simulink model "EMPlanner_cs"  (R2020a)
settings: Solver=ode5  StartTime=0.0  StopTime=55  FixedStep=1/1000  RelTol=1e-3
PreLoadFcn:
  | mbxruntime.callbacks.PreLoadFcn(bdroot);
PostLoadFcn:
  | mbxruntime.callbacks.PostLoadFcn(bdroot);
InitFcn:
  | mbxruntime.callbacks.InitFcn(bdroot);
StartFcn:
  | mbxruntime.callbacks.StartFcn(bdroot);
StopFcn:
  | mbxruntime.callbacks.StopFcn(bdroot);
model workspace: external: MAT-File .\EMPlanner_cs_hws.mat (data not in the file)
values from neighbouring files (symbols this model uses):
  c_factor = 43.75    [emplanner_init.m]
  cf = -175016    [emplanner_init.m]
  control_predict_time = 0.01    [emplanner_init.m]
  cr = -130634    [emplanner_init.m]
  dp_col = 4    [emplanner_init.m]
  dp_row = 9    [emplanner_init.m]
  dp_sample_l = 1    [emplanner_init.m]
  dp_sample_s = 15    [emplanner_init.m]
  dp_w_obs = 1e8    (= 100000000)    [emplanner_init.m]
  dp_w_ref = 20    [emplanner_init.m]
  dp_w_smooth_dddl = 10000    [emplanner_init.m]
  dp_w_smooth_ddl = 2000    [emplanner_init.m]
  dp_w_smooth_dl = 300    [emplanner_init.m]
  KD_PID_distance = 0.0    (= 0)    [emplanner_init.m]
  KD_PID_speed = 0    [emplanner_init.m]
  KI_PID_distance = 0.0    (= 0)    [emplanner_init.m]
  KI_PID_speed = 0    [emplanner_init.m]
  KP_PID_distance = 0.5    [emplanner_init.m]
  KP_PID_speed = 1.8    [emplanner_init.m]
  la = 1.265    [emplanner_init.m]
  lb = 2.947-1.265    (= 1.682)    [emplanner_init.m]
  LQR_K1 = k(:,1)'    [emplanner_init.m]
  LQR_K2 = k(:,2)'    [emplanner_init.m]
  LQR_K3 = k(:,3)'    [emplanner_init.m]
  LQR_K4 = k(:,4)'    [emplanner_init.m]
  m = 2020    [emplanner_init.m]
  path_x = [7.7742 8.77358225507 9.77170536558 10.7685522493 11.7641171228 12.7583983581 13.7513958557 14.7431100776 15.7335416918 16.7226914411 17.7105600952 18.6971484329 ... (551 elements, 551x1)]    [test_path.mat]
  path_y = [-207.8202 -207.82020006 -207.820200616 -207.820202023 -207.82020429 -207.820207237 -207.820210603 -207.820214131 -207.82021762 -207.820220941 -207.820224011 -207.820226778 ... (551 elements, 551x1)]    [test_path.mat]
  qp_referenceline_w_length = 2    [emplanner_init.m]
  qp_referenceline_w_ref = 3    [emplanner_init.m]
  qp_referenceline_w_smooth = 1    [emplanner_init.m]
  qp_referenceline_x_lb = -0.2    [emplanner_init.m]
  qp_referenceline_x_ub = 0.2    [emplanner_init.m]
  qp_referenceline_y_lb = -0.2    [emplanner_init.m]
  qp_referenceline_y_ub = 0.2    [emplanner_init.m]
  rack_displacement = [-39.14 , -37.2 , -35.29 , -33.43 , -31.6 , -29.81 , -28.06 , -26.34 , -24.66 ,      -23.01 , -21.38 , -19.79 , -18.23 , -16.69 , -15.18 , -13.7 , -12.23 , -10.8 , -9.38 , -7.98 ,     -6.61 , -5.25 , -3.91 , -2.59 , -1.29 , 0 , 1.27 , 2.54 , 3.78 , 5.02 , 6.24 , 7.46 , 8.66 ,      9.86 , 11.05 , 12.24 , 13.41 , 14.59 , 15.76 , 16.92 , 18.09 , 19.25 , 20.42 , 21.59 , 22.76 ,      23.93 , 25.11 , 26 ...(+26 chars)    [emplanner_init.m]
  right_wheel_ground = [-70 ,-67.2 , -64.4 , -61.6 , -58.8 , -56 , -53.2 , -50.4 , -47.6 , -44.8 , -42 ,      -39.2 , -36.4 , -33.6 , -30.8 , -28 , -25.2 , -22.4 , -19.6 , -16.8 , -14 , -11.2 , -8.4 , -5.6 ,      -2.8 , 0 , 2.8 , 5.6 , 8.4 , 11.2 , 14 , 16.8 , 19.6 , 22.4 , 25.2 , 28 , 30.8 , 33.6 , 36.4 ,      39.2 , 42 , 44.8 , 47.6 , 50.4 , 53.2 , 56 , 58.8 , 61.6 , 64.4 , 67.2 , 70 ]    [emplanner_init.m]
  vx_break_point = zeros(1,5000)    [emplanner_init.m]
undefined symbols (not defined in the file or in its folder): aubr, DiscIntNeverNeededParam, tablebr, vubr, warningInitialVelocity, x0
libraries: simulink x19, PreScanSimulinkLibrary x12, simulink_extras x5, Solver_SF x1
(part 8 of 9)

== matlab function EMPlanner_cs/Audi_A8_Sedan_1/decision&planning module/EM Planner/MATLAB Function2 ==
  data: x_set_gcs input; match_point_index_set output; y_set_gcs input; path_x_set_gcs input; path_y_set_gcs input; path_heading_set_gcs input; path_kappa_set_gcs input; proj_point_x_set_gcs output; proj_point_y_set_gcs output; proj_point_heading_set_gcs output; proj_point_kappa_set_gcs output
function [match_point_index_set,proj_point_x_set_gcs,proj_point_y_set_gcs,proj_point_heading_set_gcs,...
    proj_point_kappa_set_gcs] = fcn(x_set_gcs,y_set_gcs,path_x_set_gcs,path_y_set_gcs,...
    path_heading_set_gcs,path_kappa_set_gcs)
% 该函数将批量计算点在给定路径下的匹配点编号和投影点信息   
% x_set_gcs,y_set_gcs 输入点信息集合
% path_x_set_gcs,path_y_set_gcs,path_heading_set_gcs,path_kappa_set_gcs 给定路径点信息集合
% match_point_index_set 匹配点编号集合
% proj_point_x_set_gcs,proj_point_y_set_gcs,proj_point_heading_set_gcs,proj_point_kappa_set_gcs 投影点信息集合

% 假设最多有181个点需要投影
n = 181;
% 对输出进行初始化
match_point_index_set = ones(n,1) *nan; 
proj_point_x_set_gcs = ones(n,1) *nan;  proj_point_y_set_gcs = ones(n,1) *nan;
proj_point_heading_set_gcs = ones(n,1) *nan;  proj_point_kappa_set_gcs = ones(n,1) *nan;

% 寻找匹配点时 需要利用上一个周期的结果 因此定义需要利用的静态变量
persistent is_first_run;
persistent pre_match_point_index_set;
persistent pre_path_x_set_gcs; persistent pre_path_y_set_gcs; % 通过上个周期匹配点位矢判断遍历方向
persistent pre_path_heading_set_gcs; persistent pre_path_kappa_set_gcs;
persistent pre_x_set_gcs; persistent pre_y_set_gcs; % 判断相邻帧检测的是否是同一个障碍物

if isempty(is_first_run)
    is_first_run = 0;
    % 首次运行 所有待求点都从给定路径路径第一个点开始找 往前遍历 且距离连续增长上限设为50
    for i = 1:length(x_set_gcs) % 存在的点都在前面 遍历到nan至后面的点都不存在
        if isnan(x_set_gcs(i))
            break;
        end
        start_find_index = 1; forward_stable_backward = 1; increase_count_limit = 50;
        % 计算匹配点编号
        match_point_index = CalMatchPointIndex(x_set_gcs(i),y_set_gcs(i),path_x_set_gcs,...
        path_y_set_gcs,path_heading_set_gcs,path_kappa_set_gcs,start_find_index,...
        increase_count_limit, forward_stable_backward);
        % 计算投影点信息
        [proj_point_x_gcs,proj_point_y_gcs,proj_point_heading_gcs,proj_point_kappa_gcs] = ...
        CalProjPointInfo(x_set_gcs(i),y_set_gcs(i),path_x_set_gcs,path_y_set_gcs,path_heading_set_gcs,...
        path_kappa_set_gcs,match_point_index);
        % 将每个点求解信息添加到集合
        match_point_index_set(i) = match_point_index;
        proj_point_x_set_gcs(i) = proj_point_x_gcs; proj_point_y_set_gcs(i) = proj_point_y_gcs;
        proj_point_heading_set_gcs(i) = proj_point_heading_gcs; 
        proj_point_kappa_set_gcs(i) = proj_point_kappa_gcs;
    end
    % 保存该周期信息 以便下周期使用
    pre_match_point_index_set = match_point_index_set;
    pre_path_x_set_gcs = path_x_set_gcs; pre_path_y_set_gcs = path_y_set_gcs;
    pre_path_heading_set_gcs = path_heading_set_gcs; pre_path_kappa_set_gcs = path_kappa_set_gcs;
    pre_x_set_gcs = x_set_gcs; pre_y_set_gcs = y_set_gcs;
else
    % 需要使用上周期信息
    for i = 1:length(x_set_gcs)
        if isnan(x_set_gcs(i))
            break;
        end
        % 检测相邻帧是否是同一物体求解
        dis = sqrt((x_set_gcs(i)-pre_x_set_gcs(i))^2 + (y_set_gcs(i)-pre_y_set_gcs(i))^2);
        if dis > 10  % 相邻帧(相隔0.1s)同一物体距离不可能这么大
            % 说明相邻帧不是同一物体 上周期该物体已经消失在车辆的检测范围内
            % 把上周期该物体匹配点编号信息清空
            pre_match_point_index_set(i) = nan;
        end
        if isnan(pre_match_point_index_set(i))
            % 说明该物体是第一次寻找匹配点 从头开始寻找 且往前遍历
            start_find_index = 1; forward_stable_backward = 1; increase_count_limit = 50;
        else
            % 说明该物体上周期已经寻找过匹配点  判断开始寻找编号 和遍历方向
            start_find_index = pre_match_point_index_set(i); increase_count_limit = 5;
            % 提取上周期匹配点信息
            pre_match_point_x = pre_path_x_set_gcs(pre_match_point_index_set(i));
            pre_match_point_y = pre_path_y_set_gcs(pre_match_point_index_set(i));
            pre_match_point_heading = pre_path_heading_set_gcs(pre_match_point_index_set(i));
            % 通过该物体上周期匹配点位置到本周期位置向量和上周期匹配点切向量的点乘来判断遍历方向
            vector_preMatch_current = [x_set_gcs(i),y_set_gcs(i)] - [pre_match_point_x, pre_match_point_y];
            vector_tor_preMatch = [cos(pre_match_point_heading), sin(pre_match_point_heading)];
            forward_stable_backward = dot(vector_preMatch_current, vector_tor_preMatch);
        end
        % 计算匹配点编号
        match_point_index = CalMatchPointIndex(x_set_gcs(i),y_set_gcs(i),path_x_set_gcs,...
        path_y_set_gcs,path_heading_set_gcs,path_kappa_set_gcs,start_find_index,...
        increase_count_limit, forward_stable_backward);
        % 计算投影点信息
        [proj_point_x_gcs,proj_point_y_gcs,proj_point_heading_gcs,proj_point_kappa_gcs] = ...
        CalProjPointInfo(x_set_gcs(i),y_set_gcs(i),path_x_set_gcs,path_y_set_gcs,path_heading_set_gcs,...
        path_kappa_set_gcs,match_point_index);
        % 将每个点求解信息添加到集合
        match_point_index_set(i) = match_point_index;
        proj_point_x_set_gcs(i) = proj_point_x_gcs; proj_point_y_set_gcs(i) = proj_point_y_gcs;
        proj_point_heading_set_gcs(i) = proj_point_heading_gcs; 
        proj_point_kappa_set_gcs(i) = proj_point_kappa_gcs;
    end
    % 保存该周期信息 以便下周期使用
    pre_match_point_index_set = match_point_index_set;
    pre_path_x_set_gcs = path_x_set_gcs; pre_path_y_set_gcs = path_y_set_gcs;
    pre_path_heading_set_gcs = path_heading_set_gcs; pre_path_kappa_set_gcs = path_kappa_set_gcs;
    pre_x_set_gcs = x_set_gcs; pre_y_set_gcs = y_set_gcs;
end
end

== matlab function EMPlanner_cs/Audi_A8_Sedan_1/decision&planning module/EM Planner/Cartesian2Frenet/MATLAB Function4 ==
  data: ax_set input; s_dot2_set output; ay_set input; proj_heading_set input; proj_kappa_set input; l_set input; s_dot_set input; dl_set input; l_dot2_set output; ddl_set output
function [s_dot2_set,l_dot2_set,ddl_set] = fcn(ax_set,ay_set,proj_heading_set,proj_kappa_set,l_set,s_dot_set,dl_set)
%由于不知道有多少个点需要做坐标转换，设一个最大值做缓冲
n = 128;
% 输出初始化
s_dot2_set = ones(n,1)*nan;
l_dot2_set = ones(n,1)*nan;
ddl_set = ones(n,1)*nan;

for i = 1:length(l_set)
    if isnan(l_set(i))
       break;
    end
    a_h = [ax_set(i);ay_set(i)];
    n_r = [-sin(proj_heading_set(i));cos(proj_heading_set(i))];
    t_r = [cos(proj_heading_set(i));sin(proj_heading_set(i))];
    %近似认为dkr/ds 为0 简化计算
    l_dot2_set(i) = a_h'*n_r - proj_kappa_set(i) * (1 - proj_kappa_set(i) * l_set(i)) * s_dot_set(i)^2;
    s_dot2_set(i) = (1/(1 - proj_kappa_set(i) * l_set(i)))* (a_h' * t_r + 2 * proj_kappa_set(i) * dl_set(i) * s_dot_set(i)^2);
    % 要考虑加速度为0的情况
    if (s_dot2_set(i) < 1e-6)
        ddl_set(i) = 0;
    else
        ddl_set(i) = (l_dot2_set(i) - dl_set(i)*s_dot2_set(i))/(s_dot_set(i)^2);
    end
end

== matlab function EMPlanner_cs/Audi_A8_Sedan_1/decision&planning module/EM Planner/increase DP path nodes1 ==
  data: plan_start_point_s_fcs input; dp_path_s_final_set_fcs output; plan_start_point_l_fcs input; plan_start_point_dl_fcs input; plan_start_point_ddl_fcs input; dp_path_s_init_set_fcs input; dp_path_l_init_set_fcs input; dp_path_l_final_set_fcs output; dp_path_dl_final_set_fcs output; dp_path_ddl_final_set_fcs output
function [dp_path_s_final_set_fcs,dp_path_l_final_set_fcs,dp_path_dl_final_set_fcs,dp_path_ddl_final_set_fcs] = ...
    fcn(plan_start_point_s_fcs,plan_start_point_l_fcs,plan_start_point_dl_fcs,plan_start_point_ddl_fcs,dp_path_s_init_set_fcs,dp_path_l_init_set_fcs)
% 原有的动态规划的路径点太少  该函数用来增密路径点
% 输入:plan_start_point_info_fcs 规划起点信息 dp_path_info_init_set_fcs 动态规划初始点集合信息
% 输出:dp_path_info_final_set_fcs 动态规划最终点集合信息
% 原有的动态规划的路径点太少  该函数用来增密原有的动态规划得到的初始路径点
% 通过原有的规划点进行增密
% 假设增密之后横向每隔一米踩一个点
ds = 1;
% 原来路径为 规划起点-> 动态规划点1 -> 动态规划点2 -> 动态规划点3 -> 动态规划点4 -> 动态规划点5
% 增密后路径为 规划起点->(新增点->新增点->新增点)->动态规划点1->(新增点->新增点->新增点)->动态规划点2->...
% 如 规划起点-> 动态规划点1 为一个五次多项式  通过ds取多项式多个点 即为新增的点

% 假设增密之后最多200个点
n = 200;
% 输出初始化
dp_path_s_final_set_fcs = ones(n,1)*nan;dp_path_l_final_set_fcs = ones(n,1)*nan;
dp_path_dl_final_set_fcs = ones(n,1)*nan; dp_path_ddl_final_set_fcs = ones(n,1)*nan;

% 第一个五次多项式的起点为规划起点
start_s = plan_start_point_s_fcs; start_l = plan_start_point_l_fcs; 
start_dl = plan_start_point_dl_fcs; start_ddl = plan_start_point_ddl_fcs;

s_cur = []; l_cur = []; dl_cur = []; ddl_cur = []; %开辟动态数组存储所有采样点

for i = 1:length(dp_path_s_init_set_fcs)
    if isnan(dp_path_s_init_set_fcs(i))
        break;   %点不存在 退出
    end
    s_temp = []; l_temp = []; dl_temp = []; ddl_temp = []; %开辟临时动态数组存储当前循环采样点
    % 对规划起点-> 动态规划点1 -> 动态规划点2 -> 动态规划点3 -> 动态规划点4 -> 动态规划点5->...进行采样
    for j = 1:10000  % 取个较大的循环 下面通过条件break退出循环就
        s_node = start_s + ds * (j-1);   %增密后各个采样点s坐标  l,dl,ddl需要通过五次多项式计算
        if s_node < dp_path_s_init_set_fcs(i)
            s_temp = [s_temp, s_node]; % 将满足条件的增密点添加进数组
        else
            break;
        end
    end
    % % 求出五次多项式终点的边界条件
    end_s = dp_path_s_init_set_fcs(i); end_l = dp_path_l_init_set_fcs(i); end_dl = 0; end_ddl = 0;
    [a0,a1,a2,a3,a4,a5] = CalQuinticCoeffient(start_s,start_l,start_dl,start_ddl,end_s,end_l,end_dl,end_ddl);
    % 通过五次多项式求出每个采样点的l,dl,ddl
    for k = 1:length(s_temp)
        l_node = a0 + a1 * s_temp(k) + a2 * s_temp(k)^2+ a3 * s_temp(k)^3 + a4 * s_temp(k)^4 + a5 * s_temp(k)^5;
        l_temp = [l_temp,l_node];
        dl_node = a1 + 2 * a2 * s_temp(k) + 3 * a3 * s_temp(k)^2 + 4 * a4 * s_temp(k)^3 + 5 * a5 * s_temp(k)^4;
        dl_temp = [dl_temp,dl_node];
        ddl_node = 2 * a2 + 6 * a3 * s_temp(k) + 12 * a4 * s_temp(k)^2 + 20 * a5 * s_temp(k)^3;
        ddl_temp = [ddl_temp, ddl_node];
    end 
    % 将当前循环记录的采样点信息记录到总的动态数组里
    s_cur = [s_cur, s_temp]; l_cur = [l_cur, l_temp]; dl_cur = [dl_cur, dl_temp]; ddl_cur = [ddl_cur, ddl_temp];           
     % end的值赋值给start 做下一步循环
    start_s = end_s;start_l = end_l;start_dl = end_dl;start_ddl = end_ddl;
end

for i = 1:length(s_cur)
    % 防止增密之后点的个数超过最大容量
    if i > n
        break;
    end
    % 保证s坐标严格单调上升
    dp_path_s_final_set_fcs(i) = plan_start_point_s_fcs + ds * (i - 1);
%     dp_path_s_final_set_fcs(i) = s_cur(i);
    dp_path_l_final_set_fcs(i) = l_cur(i);
    dp_path_dl_final_set_fcs(i) = dl_cur(i);
    dp_path_ddl_final_set_fcs(i) = ddl_cur(i);
end
end

== matlab function EMPlanner_cs/Audi_A8_Sedan_1/decision&planning module/EM Planner/obs/MATLAB Function3 ==
  data: x_set_gcs input; match_point_index_set output; y_set_gcs input; path_x_set_gcs input; path_y_set_gcs input; path_heading_set_gcs input; path_kappa_set_gcs input; proj_point_x_set_gcs output; proj_point_y_set_gcs output; proj_point_heading_set_gcs output; proj_point_kappa_set_gcs output
function [match_point_index_set,proj_point_x_set_gcs,proj_point_y_set_gcs,proj_point_heading_set_gcs,...
    proj_point_kappa_set_gcs] = fcn(x_set_gcs,y_set_gcs,path_x_set_gcs,path_y_set_gcs,...
    path_heading_set_gcs,path_kappa_set_gcs)
% 该函数将批量计算点在给定路径下的匹配点编号和投影点信息   
% x_set_gcs,y_set_gcs 输入点信息集合
% path_x_set_gcs,path_y_set_gcs,path_heading_set_gcs,path_kappa_set_gcs 给定路径点信息集合
% match_point_index_set 匹配点编号集合
% proj_point_x_set_gcs,proj_point_y_set_gcs,proj_point_heading_set_gcs,proj_point_kappa_set_gcs 投影点信息集合

% 假设最多有181个点需要投影
n = 181;
% 对输出进行初始化
match_point_index_set = ones(n,1) *nan; 
proj_point_x_set_gcs = ones(n,1) *nan;  proj_point_y_set_gcs = ones(n,1) *nan;
proj_point_heading_set_gcs = ones(n,1) *nan;  proj_point_kappa_set_gcs = ones(n,1) *nan;

% 寻找匹配点时 需要利用上一个周期的结果 因此定义需要利用的静态变量
persistent is_first_run;
persistent pre_match_point_index_set;
persistent pre_path_x_set_gcs; persistent pre_path_y_set_gcs; % 通过上个周期匹配点位矢判断遍历方向
persistent pre_path_heading_set_gcs; persistent pre_path_kappa_set_gcs;
persistent pre_x_set_gcs; persistent pre_y_set_gcs; % 判断相邻帧检测的是否是同一个障碍物

if isempty(is_first_run)
    is_first_run = 0;
    % 首次运行 所有待求点都从给定路径路径第一个点开始找 往前遍历 且距离连续增长上限设为50
    for i = 1:length(x_set_gcs) % 存在的点都在前面 遍历到nan至后面的点都不存在
        if isnan(x_set_gcs(i))
            break;
        end
        start_find_index = 1; forward_stable_backward = 1; increase_count_limit = 50;
        % 计算匹配点编号
        match_point_index = CalMatchPointIndex(x_set_gcs(i),y_set_gcs(i),path_x_set_gcs,...
        path_y_set_gcs,path_heading_set_gcs,path_kappa_set_gcs,start_find_index,...
        increase_count_limit, forward_stable_backward);
        % 计算投影点信息
        [proj_point_x_gcs,proj_point_y_gcs,proj_point_heading_gcs,proj_point_kappa_gcs] = ...
        CalProjPointInfo(x_set_gcs(i),y_set_gcs(i),path_x_set_gcs,path_y_set_gcs,path_heading_set_gcs,...
        path_kappa_set_gcs,match_point_index);
        % 将每个点求解信息添加到集合
        match_point_index_set(i) = match_point_index;
        proj_point_x_set_gcs(i) = proj_point_x_gcs; proj_point_y_set_gcs(i) = proj_point_y_gcs;
        proj_point_heading_set_gcs(i) = proj_point_heading_gcs; 
        proj_point_kappa_set_gcs(i) = proj_point_kappa_gcs;
    end
    % 保存该周期信息 以便下周期使用
    pre_match_point_index_set = match_point_index_set;
    pre_path_x_set_gcs = path_x_set_gcs; pre_path_y_set_gcs = path_y_set_gcs;
    pre_path_heading_set_gcs = path_heading_set_gcs; pre_path_kappa_set_gcs = path_kappa_set_gcs;
    pre_x_set_gcs = x_set_gcs; pre_y_set_gcs = y_set_gcs;
else
    % 需要使用上周期信息
    for i = 1:length(x_set_gcs)
        if isnan(x_set_gcs(i))
            break;
        end
        % 检测相邻帧是否是同一物体求解
        dis = sqrt((x_set_gcs(i)-pre_x_set_gcs(i))^2 + (y_set_gcs(i)-pre_y_set_gcs(i))^2);
        if dis > 10  % 相邻帧(相隔0.1s)同一物体距离不可能这么大
            % 说明相邻帧不是同一物体 上周期该物体已经消失在车辆的检测范围内
            % 把上周期该物体匹配点编号信息清空
            pre_match_point_index_set(i) = nan;
        end
        if isnan(pre_match_point_index_set(i))
            % 说明该物体是第一次寻找匹配点 从头开始寻找 且往前遍历
            start_find_index = 1; forward_stable_backward = 1; increase_count_limit = 50;
        else
            % 说明该物体上周期已经寻找过匹配点  判断开始寻找编号 和遍历方向
            start_find_index = pre_match_point_index_set(i); increase_count_limit = 5;
            % 提取上周期匹配点信息
            pre_match_point_x = pre_path_x_set_gcs(pre_match_point_index_set(i));
            pre_match_point_y = pre_path_y_set_gcs(pre_match_point_index_set(i));
            pre_match_point_heading = pre_path_heading_set_gcs(pre_match_point_index_set(i));
            % 通过该物体上周期匹配点位置到本周期位置向量和上周期匹配点切向量的点乘来判断遍历方向
            vector_preMatch_current = [x_set_gcs(i),y_set_gcs(i)] - [pre_match_point_x, pre_match_point_y];
            vector_tor_preMatch = [cos(pre_match_point_heading), sin(pre_match_point_heading)];
            forward_stable_backward = dot(vector_preMatch_current, vector_tor_preMatch);
        end
        % 计算匹配点编号
        match_point_index = CalMatchPointIndex(x_set_gcs(i),y_set_gcs(i),path_x_set_gcs,...
        path_y_set_gcs,path_heading_set_gcs,path_kappa_set_gcs,start_find_index,...
        increase_count_limit, forward_stable_backward);
        % 计算投影点信息
        [proj_point_x_gcs,proj_point_y_gcs,proj_point_heading_gcs,proj_point_kappa_gcs] = ...
        CalProjPointInfo(x_set_gcs(i),y_set_gcs(i),path_x_set_gcs,path_y_set_gcs,path_heading_set_gcs,...
        path_kappa_set_gcs,match_point_index);
        % 将每个点求解信息添加到集合
        match_point_index_set(i) = match_point_index;
        proj_point_x_set_gcs(i) = proj_point_x_gcs; proj_point_y_set_gcs(i) = proj_point_y_gcs;
        proj_point_heading_set_gcs(i) = proj_point_heading_gcs; 
        proj_point_kappa_set_gcs(i) = proj_point_kappa_gcs;
    end
    % 保存该周期信息 以便下周期使用
    pre_match_point_index_set = match_point_index_set;
    pre_path_x_set_gcs = path_x_set_gcs; pre_path_y_set_gcs = path_y_set_gcs;
    pre_path_heading_set_gcs = path_heading_set_gcs; pre_path_kappa_set_gcs = path_kappa_set_gcs;
    pre_x_set_gcs = x_set_gcs; pre_y_set_gcs = y_set_gcs;
end
end

== matlab function EMPlanner_cs/Audi_A8_Sedan_1/decision&planning module/EM Planner/obs/Cartesian2Frenet1/MATLAB Function ==
  data: x_set_gcs input; s_set_fcs output; y_set_gcs input; path_x_set_gcs input; path_y_set_gcs input; path_heading_set_gcs input; match_point_index_set input; proj_point_x_set_gcs input; proj_point_y_set_gcs input; proj_point_heading_set_gcs input; l_set_fcs output; matchPoint_index_s_set_fcs input
function [s_set_fcs,l_set_fcs] = fun(x_set_gcs,y_set_gcs,path_x_set_gcs,path_y_set_gcs,path_heading_set_gcs,match_point_index_set,...
    proj_point_x_set_gcs,proj_point_y_set_gcs,proj_point_heading_set_gcs,matchPoint_index_s_set_fcs)
% 将函数批量将给定点的(x,y)转化成(s,l)
% 假设最多有181个点需要转换坐标
n = 181;
% 输出初始化
s_set_fcs = ones(n,1)*nan; l_set_fcs = ones(n,1)*nan;
for i = 1:length(x_set_gcs)
    if isnan(x_set_gcs(i))
        break;
    end
    s_set_fcs(i) = CalSFromOriginPoint(matchPoint_index_s_set_fcs,path_x_set_gcs,path_y_set_gcs,path_heading_set_gcs,...
                                proj_point_x_set_gcs(i),proj_point_y_set_gcs(i),match_point_index_set(i));
    vector_rh = [x_set_gcs(i),y_set_gcs(i)];
    vector_rp = [proj_point_x_set_gcs(i),proj_point_y_set_gcs(i)];
    vector_np = [-sin(proj_point_heading_set_gcs(i)),cos(proj_point_heading_set_gcs(i))];
    l_set_fcs(i) = dot(vector_rh-vector_rp, vector_np);
end
end

== matlab function EMPlanner_cs/Audi_A8_Sedan_1/decision&planning module/referenceline provider/solve heading and kappa求解给定path的heading角和曲率 ==
  data: path_x_set_gcs output; path_y_set_gcs output; path_heading_set_gcs output; path_x_set_gcs input; path_y_set_gcs input; path_kappa_set_gcs output
function [path_x_set_gcs,path_y_set_gcs,path_heading_set_gcs,path_kappa_set_gcs] = fcn(path_x_set_gcs,path_y_set_gcs)
%该函数将计算全局路径的切线方向与x轴的夹角和曲率
%输入：path_x_set_gcs,path_y_set_gcs 给定路径坐标 都是列向量
%输出：path_heading_gcs path_kappa_gcs 给定路径的heading和曲率
%输出初始化
if isrow(path_x_set_gcs)
    path_x_set_gcs = path_x_set_gcs';   % 保证为列向量
    path_y_set_gcs = path_y_set_gcs';
end
[path_heading_set_gcs,path_kappa_set_gcs] = CalHeadingAndKappa(path_x_set_gcs,path_y_set_gcs);
end

== matlab function EMPlanner_cs/Audi_A8_Sedan_1/decision&planning module/referenceline provider/MATLAB Function6 ==
  data: x_set_gcs input; match_point_index_set output; y_set_gcs input; path_x_set_gcs input; path_y_set_gcs input; path_heading_set_gcs input; path_kappa_set_gcs input; proj_point_x_set_gcs output; proj_point_y_set_gcs output; proj_point_heading_set_gcs output; proj_point_kappa_set_gcs output
function [match_point_index_set,proj_point_x_set_gcs,proj_point_y_set_gcs,proj_point_heading_set_gcs,...
    proj_point_kappa_set_gcs] = fcn(x_set_gcs,y_set_gcs,path_x_set_gcs,path_y_set_gcs,...
    path_heading_set_gcs,path_kappa_set_gcs)
% 该函数将批量计算点在给定路径下的匹配点编号和投影点信息   
% x_set_gcs,y_set_gcs 输入点信息集合
% path_x_set_gcs,path_y_set_gcs,path_heading_set_gcs,path_kappa_set_gcs 给定路径点信息集合
% match_point_index_set 匹配点编号集合
% proj_point_x_set_gcs,proj_point_y_set_gcs,proj_point_heading_set_gcs,proj_point_kappa_set_gcs 投影点信息集合

% 假设最多有181个点需要投影
n = 181;
% 对输出进行初始化
match_point_index_set = ones(n,1) *nan; 
proj_point_x_set_gcs = ones(n,1) *nan;  proj_point_y_set_gcs = ones(n,1) *nan;
proj_point_heading_set_gcs = ones(n,1) *nan;  proj_point_kappa_set_gcs = ones(n,1) *nan;

% 寻找匹配点时 需要利用上一个周期的结果 因此定义需要利用的静态变量
persistent is_first_run;
persistent pre_match_point_index_set;
persistent pre_path_x_set_gcs; persistent pre_path_y_set_gcs; % 通过上个周期匹配点位矢判断遍历方向
persistent pre_path_heading_set_gcs; persistent pre_path_kappa_set_gcs;
persistent pre_x_set_gcs; persistent pre_y_set_gcs; % 判断相邻帧检测的是否是同一个障碍物

if isempty(is_first_run)
    is_first_run = 0;
    % 首次运行 所有待求点都从给定路径路径第一个点开始找 往前遍历 且距离连续增长上限设为50
    for i = 1:length(x_set_gcs) % 存在的点都在前面 遍历到nan至后面的点都不存在
        if isnan(x_set_gcs(i))
            break;
        end
        start_find_index = 1; forward_stable_backward = 1; increase_count_limit = 50;
        % 计算匹配点编号
        match_point_index = CalMatchPointIndex(x_set_gcs(i),y_set_gcs(i),path_x_set_gcs,...
        path_y_set_gcs,path_heading_set_gcs,path_kappa_set_gcs,start_find_index,...
        increase_count_limit, forward_stable_backward);
        % 计算投影点信息
        [proj_point_x_gcs,proj_point_y_gcs,proj_point_heading_gcs,proj_point_kappa_gcs] = ...
        CalProjPointInfo(x_set_gcs(i),y_set_gcs(i),path_x_set_gcs,path_y_set_gcs,path_heading_set_gcs,...
        path_kappa_set_gcs,match_point_index);
        % 将每个点求解信息添加到集合
        match_point_index_set(i) = match_point_index;
        proj_point_x_set_gcs(i) = proj_point_x_gcs; proj_point_y_set_gcs(i) = proj_point_y_gcs;
        proj_point_heading_set_gcs(i) = proj_point_heading_gcs; 
        proj_point_kappa_set_gcs(i) = proj_point_kappa_gcs;
    end
    % 保存该周期信息 以便下周期使用
    pre_match_point_index_set = match_point_index_set;
    pre_path_x_set_gcs = path_x_set_gcs; pre_path_y_set_gcs = path_y_set_gcs;
    pre_path_heading_set_gcs = path_heading_set_gcs; pre_path_kappa_set_gcs = path_kappa_set_gcs;
    pre_x_set_gcs = x_set_gcs; pre_y_set_gcs = y_set_gcs;
else
    % 需要使用上周期信息
    for i = 1:length(x_set_gcs)
        if isnan(x_set_gcs(i))
            break;
        end
        % 检测相邻帧是否是同一物体求解
        dis = sqrt((x_set_gcs(i)-pre_x_set_gcs(i))^2 + (y_set_gcs(i)-pre_y_set_gcs(i))^2);
        if dis > 10  % 相邻帧(相隔0.1s)同一物体距离不可能这么大
            % 说明相邻帧不是同一物体 上周期该物体已经消失在车辆的检测范围内
            % 把上周期该物体匹配点编号信息清空
            pre_match_point_index_set(i) = nan;
        end
        if isnan(pre_match_point_index_set(i))
            % 说明该物体是第一次寻找匹配点 从头开始寻找 且往前遍历
            start_find_index = 1; forward_stable_backward = 1; increase_count_limit = 50;
        else
            % 说明该物体上周期已经寻找过匹配点  判断开始寻找编号 和遍历方向
            start_find_index = pre_match_point_index_set(i); increase_count_limit = 5;
            % 提取上周期匹配点信息
            pre_match_point_x = pre_path_x_set_gcs(pre_match_point_index_set(i));
            pre_match_point_y = pre_path_y_set_gcs(pre_match_point_index_set(i));
            pre_match_point_heading = pre_path_heading_set_gcs(pre_match_point_index_set(i));
            % 通过该物体上周期匹配点位置到本周期位置向量和上周期匹配点切向量的点乘来判断遍历方向
            vector_preMatch_current = [x_set_gcs(i),y_set_gcs(i)] - [pre_match_point_x, pre_match_point_y];
            vector_tor_preMatch = [cos(pre_match_point_heading), sin(pre_match_point_heading)];
            forward_stable_backward = dot(vector_preMatch_current, vector_tor_preMatch);
        end
        % 计算匹配点编号
        match_point_index = CalMatchPointIndex(x_set_gcs(i),y_set_gcs(i),path_x_set_gcs,...
        path_y_set_gcs,path_heading_set_gcs,path_kappa_set_gcs,start_find_index,...
        increase_count_limit, forward_stable_backward);
        % 计算投影点信息
        [proj_point_x_gcs,proj_point_y_gcs,proj_point_heading_gcs,proj_point_kappa_gcs] = ...
        CalProjPointInfo(x_set_gcs(i),y_set_gcs(i),path_x_set_gcs,path_y_set_gcs,path_heading_set_gcs,...
        path_kappa_set_gcs,match_point_index);
        % 将每个点求解信息添加到集合
        match_point_index_set(i) = match_point_index;
        proj_point_x_set_gcs(i) = proj_point_x_gcs; proj_point_y_set_gcs(i) = proj_point_y_gcs;
        proj_point_heading_set_gcs(i) = proj_point_heading_gcs; 
        proj_point_kappa_set_gcs(i) = proj_point_kappa_gcs;
    end
    % 保存该周期信息 以便下周期使用
    pre_match_point_index_set = match_point_index_set;
    pre_path_x_set_gcs = path_x_set_gcs; pre_path_y_set_gcs = path_y_set_gcs;
    pre_path_heading_set_gcs = path_heading_set_gcs; pre_path_kappa_set_gcs = path_kappa_set_gcs;
    pre_x_set_gcs = x_set_gcs; pre_y_set_gcs = y_set_gcs;
end
end

== matlab function EMPlanner_cs/Audi_A8_Sedan_1/decision&planning module/EM Planner/Cartesian2Frenet/MATLAB Function1 ==
  data: l_set_fcs input; sdot_set_fcs output; vx_set_gcs input; vy_set_gcs input; proj_point_heading_set_gcs input; proj_point_kappa_set_gcs input; ldot_set_fcs output; dl_set_fcs output
function [sdot_set_fcs, ldot_set_fcs, dl_set_fcs] = fun(l_set_fcs,vx_set_gcs,vy_set_gcs,proj_point_heading_set_gcs,proj_point_kappa_set_gcs)
% 该函数批量转化坐标得到    sdot_set_fcs, ldot_set_fcs, dl_set_fcs
% 假设最多有181个点需要转换坐标
n = 181;
% 输出初始化
sdot_set_fcs = ones(n,1)*nan; ldot_set_fcs = ones(n,1)*nan; dl_set_fcs = ones(n,1)*nan;

for i = 1:length(vx_set_gcs)
    if isnan(vx_set_gcs(i))
        break;
    end
    vector_vh = [vx_set_gcs(i),vy_set_gcs(i)];
    vector_tp = [cos(proj_point_heading_set_gcs(i)),sin(proj_point_heading_set_gcs(i))];
    vector_np = [-sin(proj_point_heading_set_gcs(i)),cos(proj_point_heading_set_gcs(i))];
    sdot_set_fcs(i) = (dot(vector_vh,vector_tp)) / (1-proj_point_kappa_set_gcs(i)*l_set_fcs(i));
    ldot_set_fcs(i) = dot(vector_vh,vector_np);
    if abs(sdot_set_fcs(i)) < 1e-6
        dl_set_fcs(i) = 0;
    else
        dl_set_fcs(i) = ldot_set_fcs(i) / sdot_set_fcs(i);
    end
end
end

== matlab function EMPlanner_cs/Audi_A8_Sedan_1/decision&planning module/EM Planner/Cartesian2Frenet/MATLAB Function2 ==
  data: ax_set_gcs input; sdotdot_set_fcs output; ay_set_gcs input; proj_point_heading_set_gcs input; proj_point_kappa_set_gcs input; l_set_fcs input; sdot_set_fcs input; dl_set_fcs input; ldotdot_set_fcs output; ddl_set_fcs output
function [sdotdot_set_fcs, ldotdot_set_fcs, ddl_set_fcs] = fun(ax_set_gcs,ay_set_gcs,proj_point_heading_set_gcs,proj_point_kappa_set_gcs,...
    l_set_fcs, sdot_set_fcs,dl_set_fcs)
% 该函数批量转化坐标得到    sdotdot_set_fcs, ldotdot_set_fcs, ddl_set_fcs
% 假设最多有181个点需要转换坐标
n = 181;
% 输出初始化
sdotdot_set_fcs = ones(n,1)*nan; ldotdot_set_fcs = ones(n,1)*nan; ddl_set_fcs = ones(n,1)*nan;

for i = 1:length(ax_set_gcs)
    if isnan(ax_set_gcs(i))
        break;
    end
    vector_ah = [ax_set_gcs(i),ay_set_gcs(i)];
    vector_tp = [cos(proj_point_heading_set_gcs(i)),sin(proj_point_heading_set_gcs(i))];
    vector_np = [-sin(proj_point_heading_set_gcs(i)),cos(proj_point_heading_set_gcs(i))];
    sdotdot_set_fcs(i) = (dot(vector_ah,vector_tp) + 2*proj_point_kappa_set_gcs(i)*dl_set_fcs(i)*sdot_set_fcs(i)^2) / (1-proj_point_kappa_set_gcs(i)*l_set_fcs(i));
    ldotdot_set_fcs(i) = dot(vector_ah,vector_np) - proj_point_kappa_set_gcs(i) * (1-proj_point_kappa_set_gcs(i)*l_set_fcs(i)) * sdot_set_fcs(i)^2;
    if abs(sdotdot_set_fcs(i)) < 1e-6
        ddl_set_fcs(i) = 0;
    else
        ddl_set_fcs(i) = (ldotdot_set_fcs(i) - dl_set_fcs(i) * sdotdot_set_fcs(i)) / sdot_set_fcs(i)^2;
    end
end
end

== matlab function EMPlanner_cs/Audi_A8_Sedan_1/decision&planning module/EM Planner/obs/obs filter ==
  data: host_x_gcs input; obs_x_set_final_gcs output; host_y_gcs input; host_heading_gcs input; obs_x_set_gcs input; obs_y_set_gcs input; obs_velocity_set_gcs input; obs_velocity_heading_set_gcs input; obs_y_set_final_gcs output; obs_velocity_set_final_gcs output; obs_velocity_heading_set_final_gcs output
function [obs_x_set_final_gcs,obs_y_set_final_gcs,obs_velocity_set_final_gcs,obs_velocity_heading_set_final_gcs] = ...
    fcn(host_x_gcs,host_y_gcs,host_heading_gcs,obs_x_set_gcs,obs_y_set_gcs,obs_velocity_set_gcs,obs_velocity_heading_set_gcs)
% 该函数将筛选障碍物，纵向[-10,60] 横向[-10,10]的障碍物才会被考虑
% 该函数只是一种单车道的临时办法，考虑到多车道情况，即使障碍物距离较远也应该考虑
% EM Planner完全体是多车道并行计算的，每个车道都生成参考线然后并行计算出多条轨迹，再选择最优的轨迹作为输出

% 假设最多检测到181个障碍物
n = 181;
% 输出初始化
obs_x_set_final_gcs = ones(n,1)*nan; obs_y_set_final_gcs = ones(n,1)*nan;
obs_velocity_set_final_gcs = ones(n,1)*nan; obs_velocity_heading_set_final_gcs = ones(n,1)*nan;

count = 1; % 记录符合要求障碍物个数
for i = 1:length(obs_x_set_gcs)
    if isnan(obs_x_set_gcs(i))
        break;
    end
%     纵向[-10,60] 是指车辆到障碍物  如果向量写反的 就会变成后方60m 前方10m 不符合原理
%     vector_host_obs = [host_x_gcs,host_y_gcs] - [obs_x_set_gcs(i),obs_y_set_gcs(i)];
    vector_host_obs = [obs_x_set_gcs(i),obs_y_set_gcs(i)] - [host_x_gcs,host_y_gcs];
    vector_th = [cos(host_heading_gcs),sin(host_heading_gcs)];
    vector_nh = [-sin(host_heading_gcs),cos(host_heading_gcs)];
    long_er = dot(vector_host_obs,vector_th);
    lat_er = dot(vector_host_obs,vector_nh);
    if long_er >= -10 && long_er <= 60 && abs(lat_er) <= 10
        obs_x_set_final_gcs(count) = obs_x_set_gcs(i);
        obs_y_set_final_gcs(count) = obs_y_set_gcs(i);
        obs_velocity_set_final_gcs(count) = obs_velocity_set_gcs(i);
        obs_velocity_heading_set_final_gcs(count) = obs_velocity_heading_set_gcs(i);
        count = count + 1;
    end
end
end

== matlab function EMPlanner_cs/Audi_A8_Sedan_1/decision&planning module/EM Planner/obs/Cartesian2Frenet1/MATLAB Function1 ==
  data: l_set input; s_dot_set output; vx_set input; vy_set input; proj_heading_set input; proj_kappa_set input; l_dot_set output; dl_set output
function [s_dot_set,l_dot_set,dl_set] = fcn(l_set,vx_set,vy_set,proj_heading_set,proj_kappa_set)
%该函数将计算frenet坐标系下的s_dot, l_dot, dl/ds
n = 128;
% 输出初始化
s_dot_set = ones(n,1)*nan;
l_dot_set = ones(n,1)*nan;
dl_set = ones(n,1)*nan;

for i = 1 : length(l_set)
    if isnan(l_set(i))
        break;
    end
    v_h = [vx_set(i);vy_set(i)];
    n_r = [-sin(proj_heading_set(i));cos(proj_heading_set(i))];
    t_r = [cos(proj_heading_set(i));sin(proj_heading_set(i))];
    l_dot_set(i) = v_h'*n_r;
    s_dot_set(i) = v_h'*t_r/(1 - proj_kappa_set(i)*l_set(i));
    %%%向量法做cartesian与frenet的转换要更简单，但是也有缺点，向量法必须依赖速度加速度
    %l' = l_dot/s_dot 但是如果s_dot = 0 此方法就失效了
    if abs(s_dot_set(i)) < 1e-6
        dl_set(i) = 0;
    else
        dl_set(i) = l_dot_set(i)/s_dot_set(i);
    end
end

== matlab function EMPlanner_cs/Audi_A8_Sedan_1/decision&planning module/EM Planner/obs/Cartesian2Frenet1/MATLAB Function2 ==
  data: ax_set input; s_dot2_set output; ay_set input; proj_heading_set input; proj_kappa_set input; l_set input; s_dot_set input; dl_set input; l_dot2_set output; ddl_set output
function [s_dot2_set,l_dot2_set,ddl_set] = fcn(ax_set,ay_set,proj_heading_set,proj_kappa_set,l_set,s_dot_set,dl_set)
%由于不知道有多少个点需要做坐标转换，设一个最大值做缓冲
n = 128;
% 输出初始化
s_dot2_set = ones(n,1)*nan;
l_dot2_set = ones(n,1)*nan;
ddl_set = ones(n,1)*nan;

for i = 1:length(l_set)
    if isnan(l_set(i))
       break;
    end
    a_h = [ax_set(i);ay_set(i)];
    n_r = [-sin(proj_heading_set(i));cos(proj_heading_set(i))];
    t_r = [cos(proj_heading_set(i));sin(proj_heading_set(i)];
    %近似认为dkr/ds 为0 简化计算
    l_dot2_set(i) = a_h'*n_r - proj_kappa_set(i) * (1 - proj_kappa_set(i) * l_set(i)) * s_dot_set(i)^2;
    s_dot2_set(i) = (1/(1 - proj_kappa_set(i) * l_set(i)))* (a_h' * t_r + 2 * proj_kappa_set(i) * dl_set(i) * s_dot_set(i)^2);
    % 要考虑加速度为0的情况
    if (s_dot2_set(i) < 1e-6)
        ddl_set(i) = 0;
    else
        ddl_set(i) = (l_dot2_set(i) - dl_set(i)*s_dot2_set(i))/(s_dot_set(i)^2);
    end
end

== matlab function EMPlanner_cs/Audi_A8_Sedan_1/decision&planning module/EM Planner/obs/MATLAB Function ==
  data: obs_x_set_gcs input; static_obs_x_set_gcs output; obs_y_set_gcs input; obs_velocity_set_gcs input; obs_velocity_heading_set_gcs input; static_obs_y_set_gcs output; dynamic_obs_x_set_gcs output; dynamic_obs_y_set_gcs output; dynamic_obs_vx_set_gcs output; dynamic_obs_vy_set_gcs output
function [static_obs_x_set_gcs,static_obs_y_set_gcs,dynamic_obs_x_set_gcs,dynamic_obs_y_set_gcs,...
    dynamic_obs_vx_set_gcs,dynamic_obs_vy_set_gcs] = fcn(obs_x_set_gcs,obs_y_set_gcs,obs_velocity_set_gcs,obs_velocity_heading_set_gcs)

% 该函数将分类静态障碍物和动态障碍物
% 输出初始化
n = 181;
static_obs_x_set_gcs = ones(n,1)*nan; static_obs_y_set_gcs = ones(n,1)*nan;
dynamic_obs_x_set_gcs = ones(n,1)*nan; dynamic_obs_y_set_gcs = ones(n,1)*nan;
dynamic_obs_vx_set_gcs = ones(n,1)*nan; dynamic_obs_vy_set_gcs = ones(n,1)*nan;
count_static = 1;
count_dynamic = 1;

for i = 1:length(obs_x_set_gcs)
    if isnan(obs_x_set_gcs(i))
        break;
    end
    if abs(obs_velocity_set_gcs(i)) < 0.1
        % 速度小于0.1m/s 视为静态障碍物
        static_obs_x_set_gcs(count_static) = obs_x_set_gcs(i);
        static_obs_y_set_gcs(count_static) = obs_y_set_gcs(i);
        count_static = count_static + 1;
    else
        dynamic_obs_x_set_gcs(count_dynamic) = obs_x_set_gcs(i);
        dynamic_obs_y_set_gcs(count_dynamic) = obs_y_set_gcs(i);
        dynamic_obs_vx_set_gcs(count_dynamic) = obs_velocity_set_gcs(i) * cos(obs_velocity_heading_set_gcs(i));
        dynamic_obs_vy_set_gcs(count_dynamic) = obs_velocity_set_gcs(i) * sin(obs_velocity_heading_set_gcs(i));
        count_dynamic = count_dynamic + 1;
    end
end
end

== matlab function EMPlanner_cs/Audi_A8_Sedan_1/全局路径(routine导航)模块/solve heading and kappa求解给定path的heading角和曲率 ==
  data: path_x_set_gcs output; path_y_set_gcs output; path_heading_set_gcs output; path_x_set_gcs input; path_y_set_gcs input; path_kappa_set_gcs output
function [path_x_set_gcs,path_y_set_gcs,path_heading_set_gcs,path_kappa_set_gcs] = fcn(path_x_set_gcs,path_y_set_gcs)
%该函数将计算全局路径的切线方向与x轴的夹角和曲率
%输入：path_x_set_gcs,path_y_set_gcs 给定路径坐标 都是列向量
%输出：path_heading_gcs path_kappa_gcs 给定路径的heading和曲率
%输出初始化
if isrow(path_x_set_gcs)
    path_x_set_gcs = path_x_set_gcs';   % 保证为列向量
    path_y_set_gcs = path_y_set_gcs';
end
[path_heading_set_gcs,path_kappa_set_gcs] = CalHeadingAndKappa(path_x_set_gcs,path_y_set_gcs);
end

== matlab function EMPlanner_cs/Audi_A8_Sedan_1/decision&planning module/EM Planner/calc path length and map between point and s ==
  data: path_x_set_gcs input; path_length output; path_y_set_gcs input; path_s_set_fcs output
function [path_length,path_s_set_fcs] = fcn(path_x_set_gcs,path_y_set_gcs)
% 该函数将用来计算给定路径的整个弧长 以及给定路径每个采样点到第一个采样点的弧长
n = length(path_x_set_gcs);
path_s_set_fcs = zeros(n,1);
flag = 1;
for i = 2:length(path_x_set_gcs)
    if isnan(path_x_set_gcs(i))
        flag = 0;
        break;
    end
    dis = sqrt((path_x_set_gcs(i)-path_x_set_gcs(i-1))^2 + (path_y_set_gcs(i)-path_y_set_gcs(i-1))^2);
    path_s_set_fcs(i) = path_s_set_fcs(i-1) + dis;
end

% 计算整个弧长 需要判断是遍历完推出 还是中途遇到不存在的点退出
if flag == 1
    % 正常退出
    path_length = path_s_set_fcs(end);
else
    path_length = path_s_set_fcs(i-1);
end
end

== matlab function EMPlanner_cs/Audi_A8_Sedan_1/decision&planning module/EM Planner/Frenet2Cartesian ==
  data: s_set_fcs input; x_set_gcs output; l_set_fcs input; dl_set_fcs input; ddl_set_fcs input; path_x_set_gcs input; path_y_set_gcs input; path_heading_set_gcs input; path_kappa_set_gcs input; matchPoint_index_s_set_fcs input; y_set_gcs output; heading_set_gcs output; kappa_set_gcs output
function [x_set_gcs,y_set_gcs,heading_set_gcs,kappa_set_gcs] = fcn(s_set_fcs,l_set_fcs,dl_set_fcs,ddl_set_fcs,...
    path_x_set_gcs,path_y_set_gcs,path_heading_set_gcs,path_kappa_set_gcs,matchPoint_index_s_set_fcs)
% 该函数将批量将(s,l) 转化成 (x,y)
% s_set_fcs,l_set_fcs,dl_set_fcs,ddl_set_fcs 转换点 自然坐标系信息
% path_x_set_gcs,path_y_set_gcs,path_heading_set_gcs,path_kappa_set_gcs 给定路径采样点信息
% matchPoint_index_s_set_fcs 给定路径采样点s坐标集合
% 假设最多有181个点需要转换
n = 181;
% 输出初始化
x_set_gcs = ones(n,1)*nan; y_set_gcs = ones(n,1)*nan; heading_set_gcs = ones(n,1)*nan; kappa_set_gcs = ones(n,1)*nan;
for i = 1:length(s_set_fcs)
    if isnan(s_set_fcs(i))
        break;
    end
    % 求出该点在给定路径采样点上 投影点的信息
    [proj_point_x_gcs,proj_point_y_gcs,proj_point_heading_gcs,proj_point_kappa_gcs] = ...
                CalProjPointInfoFromFrenet(s_set_fcs(i),path_x_set_gcs,path_y_set_gcs,path_heading_set_gcs,...
                                                path_kappa_set_gcs,matchPoint_index_s_set_fcs);
    x_set_gcs(i) = proj_point_x_gcs - l_set_fcs(i) * sin(proj_point_heading_gcs);
    y_set_gcs(i) = proj_point_y_gcs + l_set_fcs(i) * cos(proj_point_heading_gcs);
    heading_set_gcs(i) = proj_point_heading_gcs + atan(dl_set_fcs(i)/(1-proj_point_kappa_gcs*l_set_fcs(i)));
    k1 = ddl_set_fcs(i) + proj_point_kappa_gcs * dl_set_fcs(i) * tan(heading_set_gcs(i)-proj_point_heading_gcs);
    k2 = (cos(heading_set_gcs(i)-proj_point_heading_gcs))^2 / (1 - proj_point_kappa_gcs*l_set_fcs(i));
    k3 = cos(heading_set_gcs(i)-proj_point_heading_gcs) / (1 - proj_point_kappa_gcs*l_set_fcs(i));
    kappa_set_gcs(i) = (k1 * k2 + proj_point_kappa_gcs) * k3;
end
end

== matlab function EMPlanner_cs/Audi_A8_Sedan_1/decision&planning module/EM Planner/path and speed merge ==
  data: s input; trajectory_x output; s_dot input; s_dot2 input; relative_time input; current_time input; path_s input; trajectory_x_init input; trajectory_y_init input; trajectory_heading_init input; trajectory_kappa_init input; trajectory_y output; trajectory_heading output; trajectory_kappa output; trajectory_speed output; trajectory_accel output; trajectory_time output
function [trajectory_x,trajectory_y,trajectory_heading,trajectory_kappa,trajectory_speed,trajectory_accel,trajectory_time] = ...
    fcn(s,s_dot,s_dot2,relative_time,current_time,path_s,trajectory_x_init,trajectory_y_init,trajectory_heading_init,trajectory_kappa_init)
% 该函数将合并path和speed
% 由于path 是 60个点，speed 有 401个点，合并后，path和speed有401个点，因此需要做插值
n = 401;
trajectory_x = zeros(n,1);
trajectory_y = zeros(n,1);
trajectory_heading = zeros(n,1);
trajectory_kappa = zeros(n,1);
trajectory_speed = zeros(n,1);

trajectory_accel = zeros(n,1);
index = 1;
% 由于trajectory_x_init中不是所有的值都有效，(有nan) 所以要找到有效值的范围
while ~isnan(trajectory_x_init(index)) 
    index = index + 1;
end
index = index - 1;
trajectory_time = zeros(n,1);
for i = 1:length(trajectory_heading_init)-1
    trajectory_heading_init(i+1) = trajectory_heading_init(i) + sin(trajectory_heading_init(i+1)-trajectory_heading_init(i));
end
for i = 1:n-1
    %interp1 线性插值
    % 若 x = [1,2] y = [3,4]
    %interp1(x,y,1.5) 会得到3.5
    %interp1 的缺点是 在端点或超过端点的，结果为nan
    % interp1(x,y,2) 不会等于4 而是会等于nan
    % interp1(x,y,6) 也会等于nan，所以在端点处要单独处理
    trajectory_x(i) = interp1(path_s(1:index),trajectory_x_init(1:index),s(i));
    trajectory_y(i) = interp1(path_s(1:index),trajectory_y_init(1:index),s(i));
    trajectory_heading(i) = interp1(path_s(1:index),trajectory_heading_init(1:index),s(i));
    trajectory_kappa(i) = interp1(path_s(1:index),trajectory_kappa_init(1:index),s(i));
    trajectory_time(i) = relative_time(i) + current_time;%速度规划会得到相对时间，转换成绝对时间
    trajectory_speed(i) = s_dot(i);
    trajectory_accel(i) = s_dot2(i);
end
% 端点单独处理
trajectory_x(end) = trajectory_x_init(end);
trajectory_y(end) = trajectory_y_init(end);
trajectory_heading(end) = trajectory_heading_init(end);
trajectory_kappa(end) = trajectory_kappa_init(end);
trajectory_time(end) = relative_time(end) + current_time;
trajectory_speed(end) = s_dot(end);
trajectory_accel(end) = s_dot2(end);

== matlab function EMPlanner_cs/Audi_A8_Sedan_1/decision&planning module/EM Planner/increase st point count ==
  data: s_init input; s output; s_dot_init input; s_dot2_init input; relative_time_init input; s_dot output; s_dot2 output; relative_time output
function [s,s_dot,s_dot2,relative_time] = fcn(s_init,s_dot_init,s_dot2_init,relative_time_init)
%该函数将增密s s_dot s_dot2
% 为什么需要增密，因为控制的执行频率是规划的10倍，轨迹点如果不够密，必然会导致规划效果不好
% 但是若在速度二次规划中点取的太多，会导致二次规划的矩阵规模太大计算太慢
% 所以方法是在二次规划中选取少量的点优化完毕后，在用此函数增密
T = relative_time_init(end);
n = 401;
dt = T/(n-1);
s = zeros(n,1);
s_dot = zeros(n,1);
s_dot2 = zeros(n,1);
relative_time = zeros(n,1);
for i = 1:n
    current_t = (i-1)*dt;
    for j = 1:length(relative_time_init)-1
        if relative_time_init(j) <= current_t && relative_time_init(j+1) > current_t
            break;
        end
    end
    x = current_t - relative_time_init(j);
    s(i) = s_init(j) + s_dot_init(j)*x + (1/3)*s_dot2_init(j)*x^2 + (1/6)*s_dot2_init(j+1)*x^2; 
    s_dot(i) = s_dot_init(j) + 0.5*s_dot2_init(j)*x + 0.5*s_dot2_init(j+1)*x;
    s_dot2(i) = s_dot2_init(j) + (s_dot2_init(j+1) - s_dot2_init(j))*x/(relative_time_init(j+1) - relative_time_init(j));
    relative_time(i) = current_t;
end

== matlab function EMPlanner_cs/Audi_A8_Sedan_1/decision&planning module/EM Planner/stitch trajectory ==
  data: trajectory_x input; trajectory_x_final output; trajectory_y input; trajectory_heading input; trajectory_kappa input; trajectory_speed input; trajectory_accel input; trajectory_time input; stitch_x input; stitch_y input; stitch_heading input; stitch_kappa input; stitch_speed input; stitch_accel input; stitch_time input; trajectory_y_final output; trajectory_heading_final output; trajectory_kappa_final output; trajectory_speed_final output; trajectory_accel_final output; trajectory_time_final output
function [trajectory_x_final,trajectory_y_final,trajectory_heading_final,trajectory_kappa_final,...
          trajectory_speed_final,trajectory_accel_final,trajectory_time_final] = fcn(trajectory_x,...
          trajectory_y,trajectory_heading,trajectory_kappa,trajectory_speed,trajectory_accel,trajectory_time,...
          stitch_x,stitch_y,stitch_heading,stitch_kappa,stitch_speed,stitch_accel,stitch_time)
% 轨迹拼接，把stitch trajectory 拼到规划完成的轨迹上
n = 401 + 20;
trajectory_x_final = zeros(n,1);
trajectory_y_final = zeros(n,1);
trajectory_heading_final = zeros(n,1);
trajectory_kappa_final = zeros(n,1);
trajectory_speed_final = zeros(n,1);
trajectory_accel_final = zeros(n,1);
trajectory_time_final = zeros(n,1);

trajectory_x_final = [stitch_x;trajectory_x];
trajectory_y_final = [stitch_y;trajectory_y];
trajectory_heading_final = [stitch_heading;trajectory_heading];
trajectory_kappa_final = [stitch_kappa;trajectory_kappa];
trajectory_speed_final = [stitch_speed;trajectory_speed];
trajectory_accel_final = [stitch_accel;trajectory_accel];
trajectory_time_final = [stitch_time;trajectory_time];

== matlab function EMPlanner_cs/Audi_A8_Sedan_1/decision&planning module/EM Planner/path decision with dynamic planning(dp) ==
  data: obs_s_set_fcs input; dpPath_s_init_set_fcs output; obs_l_set_fcs input; plan_startPoint_s_fcs input; plan_startPoint_l_fcs input; plan_startPoint_dl_fcs input; plan_startPoint_ddl_fcs input; w_obs input; w_smooth_dl input; w_smooth_ddl input; w_smooth_dddl input; w_ref input; row input; col input; sample_s input; sample_l input; dpPath_l_init_set_fcs output
function [dpPath_s_init_set_fcs,dpPath_l_init_set_fcs] = fcn(obs_s_set_fcs,obs_l_set_fcs,plan_startPoint_s_fcs,...
    plan_startPoint_l_fcs,plan_startPoint_dl_fcs,plan_startPoint_ddl_fcs,...
         w_obs,w_smooth_dl,w_smooth_ddl,w_smooth_dddl,w_ref,row,col,sample_s,sample_l)
% 该函数将通过动态规划出一条初始路径来实现避障
% obs_s_set_fcs,obs_l_set_fcs 障碍物坐标信息
% plan_startPoint_s_fcs,plan_startPoint_l_fcs,plan_startPoint_dl_fcs,plan_startPoint_ddl_fcs 规划起点信息
%  w_obs,w_smooth_dl,w_smooth_ddl,w_smooth_dddl,w_ref 动态规划权重参数
% 采样点的行 列 行间距 列间距  行数必须为技术  且中间行的点需要刚好在s轴上
mid_row = (row+1)/2;
% dpPath_s_init_set_fcs,dpPath_l_init_set_fcs  暂时不包括规划起点
% 输出初始化
% 假设最多取20列采样点
max_col = 20;
dpPath_s_init_set_fcs = ones(max_col,1) * nan; dpPath_l_init_set_fcs = ones(max_col,1) * nan;
node_minCost_set = ones(row,col) * inf; % 用来记录自车从规划起点到每个采样点的最小代价
preCol_bestRow_set = zeros(row, col); % 用来记录到达该采样点最优路径前一列的行号   第一列采样点前一列最优行号视为0

% 首先计算规划起点到第一列所有采样点的代价
for i = 1:row
    pre_col_node_s_fcs = plan_startPoint_s_fcs; pre_col_node_l_fcs = plan_startPoint_l_fcs;
    pre_col_node_dl_fcs = plan_startPoint_dl_fcs; pre_col_node_ddl_fcs = plan_startPoint_ddl_fcs;
    cur_col_node_s_fcs = plan_startPoint_s_fcs + sample_s;
    cur_col_node_l_fcs = (mid_row - i) * sample_l;
    cur_col_node_dl_fcs = 0; cur_col_node_ddl_fcs = 0;
    node_minCost_set(i,1) = CalNeighbourColPointCost(pre_col_node_s_fcs,pre_col_node_l_fcs,pre_col_node_dl_fcs,pre_col_node_ddl_fcs,...
    cur_col_node_s_fcs, cur_col_node_l_fcs,cur_col_node_dl_fcs,cur_col_node_ddl_fcs, w_obs,w_smooth_dl,w_smooth_ddl,...
    w_smooth_dddl,w_ref,obs_s_set_fcs,obs_l_set_fcs,sample_s);
end

% 再计算规划起点到后续列所有采样点的最小代价 以及最优轨迹行数
% 一列一列的往后遍历
for j = 2:col
    for i = 1:row
        %遍历当前列所有行
        cur_col = j;
        cur_col_node_s_fcs = plan_startPoint_s_fcs + cur_col * sample_s;
        cur_col_node_l_fcs = (mid_row - i) * sample_l;
        cur_col_node_dl_fcs = 0; cur_col_node_ddl_fcs = 0;
        % 求解前一列所有行采样点到当前列当前行采样点的代价
        for k = 1:row
            % 遍历前一列所有行
            pre_col = j - 1;
            pre_col_node_s_fcs = plan_startPoint_s_fcs + pre_col * sample_s;
            pre_col_node_l_fcs = (mid_row - k) * sample_l;
            pre_col_node_dl_fcs = 0; pre_col_node_ddl_fcs = 0;
            % 前一列当前行采样点到当前列当前行采样点的代价
            cost = CalNeighbourColPointCost(pre_col_node_s_fcs,pre_col_node_l_fcs,pre_col_node_dl_fcs,pre_col_node_ddl_fcs,...
                cur_col_node_s_fcs, cur_col_node_l_fcs,cur_col_node_dl_fcs,cur_col_node_ddl_fcs, w_obs,w_smooth_dl,w_smooth_ddl,...
                w_smooth_dddl,w_ref,obs_s_set_fcs,obs_l_set_fcs,sample_s);
            cost = cost + node_minCost_set(k,pre_col);
            % 通过比较 最终将最小代价填充进数组
            if cost < node_minCost_set(i,cur_col)
                node_minCost_set(i,cur_col) = cost;
                preCol_bestRow_set(i,cur_col) = k;
            end
        end
    end
end

% 计算最后一列最优路径点是哪个  亦即是最终目标点
% 即计算数组node_minCost_set最后一列对应行数
lastCol_bestRow = 0;
minCost = inf;
for i = 1:row
    if node_minCost_set(i,end) < minCost
        lastCol_bestRow = i;
        minCost = node_minCost_set(i,end);
    end
end
best_row_set = zeros(col,1); best_row_set(end) = lastCol_bestRow;
best_row = lastCol_bestRow;
% 再计算到达最后一列最优路径点 前面所经历过的轨迹行数
for j = col:-1:2
    best_row = preCol_bestRow_set(best_row,j);
    best_row_set(j-1) = best_row;
end

% 根据最优路径行号 求解最优路径采样点坐标
for j = 1:col
    if j > max_col
        break;
    end
    dpPath_s_init_set_fcs(j) = plan_startPoint_s_fcs + j * sample_s;
    dpPath_l_init_set_fcs(j) = (mid_row - best_row_set(j)) * sample_l;
end
end
